simulink model "AS5600"  (R2018a)
settings: Solver=FixedStepAuto  StartTime=0.0  StopTime=inf  RelTol=1e-3  EnableMultiTasking=on
libraries: arduinolib x5, dspswit3 x1, commsynccomp2 x1, simulink x1
settings Model: SimulationMode=external  ExtModeTrigDuration=2  Creator=kanes  LastModifiedBy=kanes
settings OptimizationCC: EnhancedBackFolding=on  PassReuseOutputArgsThreshold=0  MaxStackSize=64  OptimizeBlockOrder=speed  DifferentSizesBufferReuse=on  OptimizationCustomize=off
settings DebuggingCC: ParameterTunabilityLossMsg=error
settings HardwareCC: ProdBitPerInt=16  ProdBitPerPointer=16  ProdBitPerSizeT=16  ProdBitPerPtrDiffT=16  ProdLargestAtomicFloat=None  ProdWordSize=8  ProdHWDeviceType=Atmel->AVR  UseEmbeddedCoderFeatures=off  UseSimulinkCoderFeatures=off
settings SFSimCC: MATLABDynamicMemAlloc=off
settings RTWCC: SystemTargetFile=ert.tlc  HardwareBoard=Arduino Uno  TLCOptions=-aInlineSetEventsForThisBaseRateFcn=TLC_FALSE -aSuppressMultiTaskScheduler=TLC_FALSE -aRateBasedStepFcn=1  TemplateMakefile=ert_default_tmf  RTWVerbose=off  Toolchain=Arduino AVR  BuildConfiguration=Faster Runs
settings CodeAppCC: ForceParamTrailComments=on  OperatorAnnotations=on  MangleLength=10
settings ERTTargetCC: ERTCustomFileBanners=off  SupportContinuousTime=on  SupportNonInlinedSFcns=on  RemoveResetFunc=off  SupportVariableSizeSignals=on  ModelStepFunctionPrototypeControlCompliant=off  ExtMode=on  ExtModeTransport=6  ExtModeMexFile=ext_serial_win32_comm_leonardo  ExtModeMexArgs=0 8 115200  ERTSrcFileBannerTemplate=codertarget_code_template.cgt  ERTHdrFileBannerTemplate=codertarget_code_template.cgt  ERTDataSrcFileTemplate=codertarget_code_template.cgt  ERTDataHdrFileTemplate=codertarget_code_template.cgt

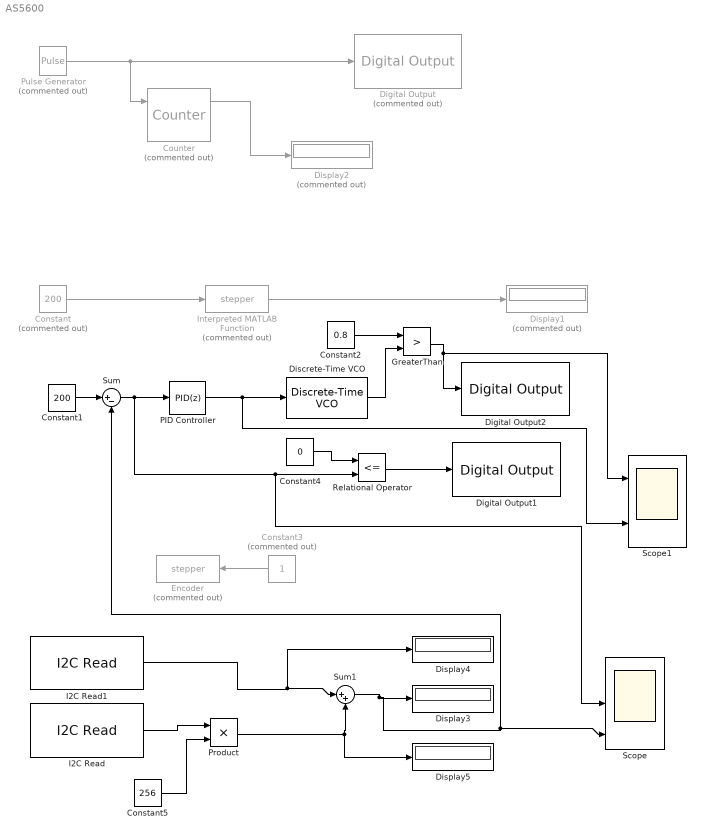
== system AS5600 ==
  Constant : Constant  Commented=on  Value=200
  Constant1 : Constant  Value=200
  Constant2 : Constant  Value=0.8
  Constant3 : Constant  Commented=on
  Constant4 : Constant  Value=0
  Constant5 : Constant  Value=256
  Counter : dspswit3/Counter  Commented=on  Direction=Up  CountEvent=Rising edge  CounterSize=User defined  MaxCount=255  InitialCount=0  Output=Count and Hit  HitValue=32  ResetInput=on  SamplesPerFrame=1  Ts=1  CntDtype=double  HitDtype=Logical
  Digital Output : arduinolib/Digital Output  Commented=on  pinNumber=13  blockPlatform=arduino
  Digital Output1 : arduinolib/Digital Output  pinNumber=4  blockPlatform=arduino
  Digital Output2 : arduinolib/Digital Output  pinNumber=3  blockPlatform=arduino
  Discrete-Time VCO : commsynccomp2/Discrete-Time VCO  Ac=1  Fc=10  Kc=1  Ph=0  ts=0.001
      settings: SourceProductName=Communications System Toolbox  SourceProductBaseCode=CM
  Display1 : Display  Commented=on
  Display2 : Display  Commented=on
  Display3 : Display
  Display4 : Display
  Display5 : Display
  Encoder : MATLABFcn  Commented=on  MATLABFcn=stepper  OutputSignalType=real
  GreaterThan : RelationalOperator  Operator=>  OutDataTypeStr=boolean  RndMeth=Simplest
  I2C Read : arduinolib/I2C Read  SlaveAddress_=hex2dec( '36' )  RegisterAddressEnable=on  RegisterAddress_=hex2dec( '0E' )  Datatype=uint8  ByteOrder=Big Endian  Datalength_=1  SampleTime_=0.001  blockPlatform=arduino
      settings: SourceProductName=Simulink Support Package for Arduino Hardware  SourceProductBaseCode=ARDUINO
  I2C Read1 : arduinolib/I2C Read  SlaveAddress_=hex2dec( '36' )  RegisterAddressEnable=on  RegisterAddress_=hex2dec( '0F' )  Datatype=uint8  ByteOrder=Big Endian  Datalength_=1  SampleTime_=0.001  blockPlatform=arduino
      settings: SourceProductName=Simulink Support Package for Arduino Hardware  SourceProductBaseCode=ARDUINO
  Interpreted MATLAB Function : MATLABFcn  Commented=on  MATLABFcn=stepper  OutputSignalType=real
  PID Controller : simulink/Continuous/PID Controller  Controller=PID  TimeDomain=Discrete-time  SampleTime=-1  IntegratorMethod=Forward Euler  FilterMethod=Forward Euler  Form=Parallel  UseFilter=on  ControllerParametersSource=internal  P=500  I=100  D=1  N=100  InitialConditionSource=internal  InitialConditionForIntegrator=0  InitialConditionForFilter=0  ExternalReset=none  LimitOutput=on  UpperSaturationLimit=1  LowerSaturationLimit=0  LinearizeAsGain=on  AntiWindupMode=none  Kb=1  TrackingMode=off  Kt=1  PParamMin=[]  PParamMax=[]  IParamMin=[]  IParamMax=[]  DParamMin=[]  DParamMax=[]  NParamMin=[]  NParamMax=[]  KbParamMin=[]  KbParamMax=[]  KtParamMin=[]  KtParamMax=[]  POutMin=[]  POutMax=[]  IOutMin=[]  IOutMax=[]  DOutMin=[]  DOutMax=[]  NOutMin=[]  NOutMax=[]  KbOutMin=[]  KbOutMax=[]  KtOutMin=[]  KtOutMax=[]  IntegratorOutMin=[]  IntegratorOutMax=[]  FilterOutMin=[]  FilterOutMax=[]  SumOutMin=[]  SumOutMax=[]  SumI1OutMin=[]  SumI1OutMax=[]  SumI2OutMin=[]  SumI2OutMax=[]  SumI3OutMin=[]  SumI3OutMax=[]  SumDOutMin=[]  SumDOutMax=[]  SaturationOutMin=[]  SaturationOutMax=[]  IntegratorContinuousStateAttributes=''  IntegratorStateMustResolveToSignalObject=off  IntegratorRTWStateStorageClass=Auto  FilterContinuousStateAttributes=''  FilterStateMustResolveToSignalObject=off  FilterRTWStateStorageClass=Auto  DifferentiatorICPrevScaledInput=0  DifferentiatorOutMin=[]  DifferentiatorOutMax=[]  FilterDiffOutCoefMin=[]  FilterDiffOutCoefMax=[]  SumDenOutMin=[]  SumDenOutMax=[]  SumNumOutMin=[]  SumNumOutMax=[]  ReciprocalOutMin=[]  ReciprocalOutMax=[]  DivideOutMin=[]  DivideOutMax=[]  TunerSelectOption=Transfer Function Based (PID Tuner App)
  Product : Product
  Pulse Generator : DiscretePulseGenerator  Commented=on  Period=10  SampleTime=0.1
  Relational Operator : RelationalOperator  Operator=<=  OutDataTypeStr=boolean  RndMeth=Simplest
  Scope : Scope  NumInputPorts=3
  Scope1 : Scope  NumInputPorts=2
  Sum : Sum  Inputs=|+-
  Sum1 : Sum  Inputs=|++
  wires:
  Pulse Generator/1 -> Counter/1, Digital Output/1
  Interpreted MATLAB Function/1 -> Display1/1
  Counter/1 -> Display2/1
  Constant/1 -> Interpreted MATLAB Function/1
  Constant1/1 -> Sum/1
  Sum/1 -> Scope/2, Relational Operator/2, PID Controller/1
  PID Controller/1 -> Discrete-Time VCO/1, Scope1/2
  Constant3/1 -> Encoder/1
  Constant4/1 -> Relational Operator/1
  Relational Operator/1 -> Digital Output1/1
  GreaterThan/1 -> Scope1/1, Digital Output2/1
  Discrete-Time VCO/1 -> GreaterThan/2
  Constant2/1 -> GreaterThan/1
  I2C Read1/1 -> Sum1/1, Display4/1
  Sum1/1 -> Scope/3, Sum/2, Display3/1
  Product/1 -> Sum1/2, Display5/1
  I2C Read/1 -> Product/1
  Constant5/1 -> Product/2
